simulink model "Scenario_Analysis_Simu"  (R2023b)
settings: Solver=VariableStepAuto  StartTime=0.0  StopTime=1  RelTol=1e-3
values from neighbouring files (symbols this model uses):
  X_init = P.X(1)    [Scenario_Analysis_Main.m]
  X_pos = P.X(i)    [Scenario_Analysis_Main.m]
  Y_init = P.Y(1)    [Scenario_Analysis_Main.m]
  Y_pos = P.Y(i)    [Scenario_Analysis_Main.m]
  Z_init = P.Z(1)    [Scenario_Analysis_Main.m]
  Z_pos = P.Z(i)    [Scenario_Analysis_Main.m]
settings Model: Creator=Dell  LastModifiedBy=Dell

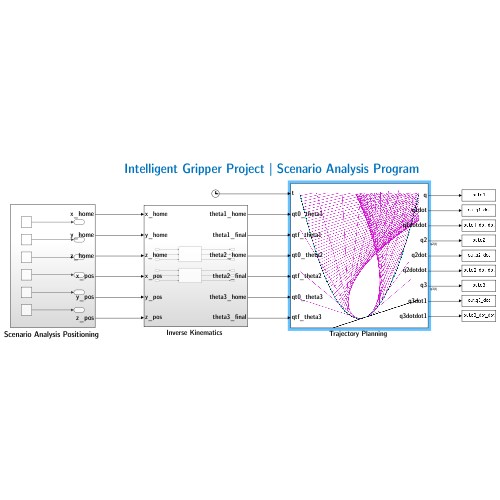
[thumbnail: Simulink's stored preview of the top-level diagram]
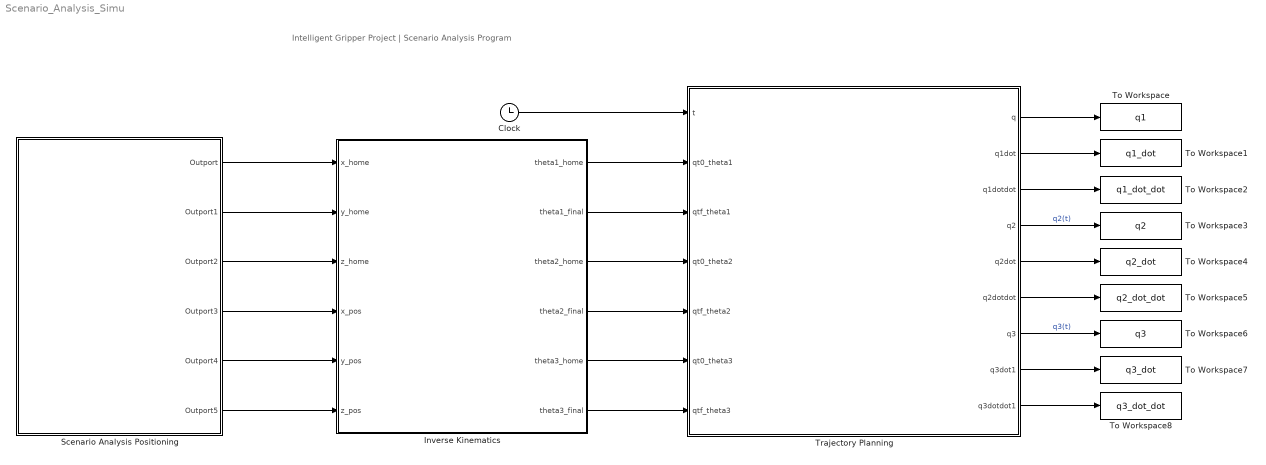
== system Scenario_Analysis_Simu ==
  note: Intelligent Gripper Project | Scenario Analysis Program
  Clock : Clock
      settings: Decimation=5
  "Inverse Kinematics " : Subsystem
  "Scenario Analysis Positioning " : Subsystem
  To Workspace : ToWorkspace  VariableName=q1  SampleTime=-1
  To Workspace1 : ToWorkspace  VariableName=q1_dot  SampleTime=-1
  To Workspace2 : ToWorkspace  VariableName=q1_dot_dot  SampleTime=-1
  To Workspace3 : ToWorkspace  VariableName=q2  SampleTime=-1
  To Workspace4 : ToWorkspace  VariableName=q2_dot  SampleTime=-1
  To Workspace5 : ToWorkspace  VariableName=q2_dot_dot  SampleTime=-1
  To Workspace6 : ToWorkspace  VariableName=q3  SampleTime=-1
  To Workspace7 : ToWorkspace  VariableName=q3_dot  SampleTime=-1
  To Workspace8 : ToWorkspace  VariableName=q3_dot_dot  SampleTime=-1
  "Trajectory Planning " : Subsystem
      mask Display: image('kisspng-caustic-tschirnhausen-cubic-curve-nephroid-parabol-caustique-wikipdia-5c6cdcbe1d93b4.9550090715506382701212.png');
  wires:
  "Inverse Kinematics "/5(theta3_home) -> "Trajectory Planning "/6(qt0_theta3)
  "Scenario Analysis Positioning "/2(Outport1) -> "Inverse Kinematics "/2(y_home)
  "Scenario Analysis Positioning "/3(Outport2) -> "Inverse Kinematics "/3(z_home)
  "Inverse Kinematics "/1(theta1_home) -> "Trajectory Planning "/2(qt0_theta1)
  "Inverse Kinematics "/2(theta1_final) -> "Trajectory Planning "/3(qtf_theta1)
  "Scenario Analysis Positioning "/1(Outport) -> "Inverse Kinematics "/1(x_home)
  "Inverse Kinematics "/6(theta3_final) -> "Trajectory Planning "/7(qtf_theta3)
  "Inverse Kinematics "/4(theta2_final) -> "Trajectory Planning "/5(qtf_theta2)
  "Scenario Analysis Positioning "/6(Outport5) -> "Inverse Kinematics "/6(z_pos)
  "Inverse Kinematics "/3(theta2_home) -> "Trajectory Planning "/4(qt0_theta2)
  "Scenario Analysis Positioning "/5(Outport4) -> "Inverse Kinematics "/5(y_pos)
  "Scenario Analysis Positioning "/4(Outport3) -> "Inverse Kinematics "/4(x_pos)
  Clock/1 -> "Trajectory Planning "/1(t)
  "Trajectory Planning "/1(q) -> To Workspace/1
  "Trajectory Planning "/2(q1dot) -> To Workspace1/1
  "Trajectory Planning "/3(q1dotdot) -> To Workspace2/1
  "Trajectory Planning "/4(q2) -> To Workspace3/1  "q2(t)"
  "Trajectory Planning "/5(q2dot) -> To Workspace4/1
  "Trajectory Planning "/6(q2dotdot) -> To Workspace5/1
  "Trajectory Planning "/7(q3) -> To Workspace6/1  "q3(t)"
  "Trajectory Planning "/8(q3dot1) -> To Workspace7/1
  "Trajectory Planning "/9(q3dotdot1) -> To Workspace8/1

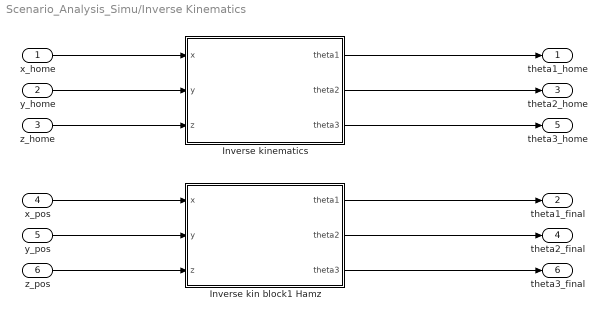
== system Scenario_Analysis_Simu/Inverse Kinematics  ==
  x_home : Inport
  y_home : Inport  Port=2
  z_home : Inport  Port=3
  x_pos : Inport  Port=4
  y_pos : Inport  Port=5
  z_pos : Inport  Port=6
  "Inverse kin block1 Hamz " : MATLAB Function  TreatAsAtomicUnit=on
  Inverse kinematics : MATLAB Function  TreatAsAtomicUnit=on
  theta1_home : Outport
  theta1_final : Outport  Port=2
  theta2_home : Outport  Port=3
  theta2_final : Outport  Port=4
  theta3_home : Outport  Port=5
  theta3_final : Outport  Port=6
  wires:
  z_home/1 -> Inverse kinematics/3(z)
  "Inverse kin block1 Hamz "/3(theta3) -> theta3_final/1
  y_home/1 -> Inverse kinematics/2(y)
  Inverse kinematics/1(theta1) -> theta1_home/1
  Inverse kinematics/3(theta3) -> theta3_home/1
  "Inverse kin block1 Hamz "/2(theta2) -> theta2_final/1
  x_home/1 -> Inverse kinematics/1(x)
  x_pos/1 -> "Inverse kin block1 Hamz "/1(x)
  Inverse kinematics/2(theta2) -> theta2_home/1
  y_pos/1 -> "Inverse kin block1 Hamz "/2(y)
  z_pos/1 -> "Inverse kin block1 Hamz "/3(z)
  "Inverse kin block1 Hamz "/1(theta1) -> theta1_final/1

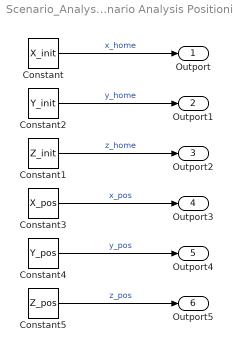
== system Scenario_Analysis_Simu/Scenario Analysis Positioning  ==
  Constant : Constant  Value=X_init
  Constant1 : Constant  Value=Z_init
  Constant2 : Constant  Value=Y_init
  Constant3 : Constant  Value=X_pos
  Constant4 : Constant  Value=Y_pos
  Constant5 : Constant  Value=Z_pos
  Outport : Outport
  Outport1 : Outport  Port=2
  Outport2 : Outport  Port=3
  Outport3 : Outport  Port=4
  Outport4 : Outport  Port=5
  Outport5 : Outport  Port=6
  wires:
  Constant/1 -> Outport/1  "x_home"
  Constant2/1 -> Outport1/1  "y_home"
  Constant3/1 -> Outport3/1  "x_pos"
  Constant4/1 -> Outport4/1  "y_pos"
  Constant5/1 -> Outport5/1  "z_pos"
  Constant1/1 -> Outport2/1  "z_home"

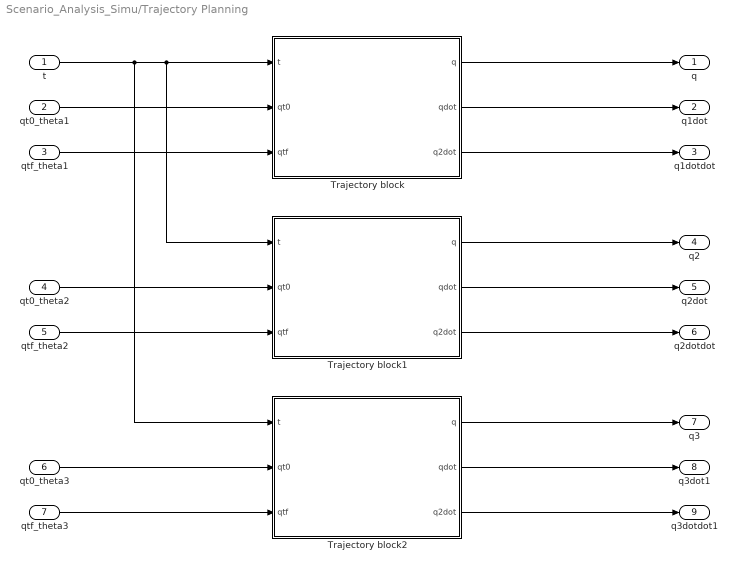
== system Scenario_Analysis_Simu/Trajectory Planning  ==
  t : Inport
  qt0_theta1 : Inport  Port=2
  qtf_theta1 : Inport  Port=3
  qt0_theta2 : Inport  Port=4
  qtf_theta2 : Inport  Port=5
  qt0_theta3 : Inport  Port=6
  qtf_theta3 : Inport  Port=7
  Trajectory block : MATLAB Function  TreatAsAtomicUnit=on
  Trajectory block1 : MATLAB Function  TreatAsAtomicUnit=on
  Trajectory block2 : MATLAB Function  TreatAsAtomicUnit=on
  q : Outport
  q1dot : Outport  Port=2
  q1dotdot : Outport  Port=3
  q2 : Outport  Port=4
  q2dot : Outport  Port=5
  q2dotdot : Outport  Port=6
  q3 : Outport  Port=7
  q3dot1 : Outport  Port=8
  q3dotdot1 : Outport  Port=9
  wires:
  qt0_theta1/1 -> Trajectory block/2(qt0)
  qtf_theta1/1 -> Trajectory block/3(qtf)
  qt0_theta2/1 -> Trajectory block1/2(qt0)
  qtf_theta2/1 -> Trajectory block1/3(qtf)
  t/1 -> Trajectory block2/1(t), Trajectory block1/1(t), Trajectory block/1(t)
  qt0_theta3/1 -> Trajectory block2/2(qt0)
  qtf_theta3/1 -> Trajectory block2/3(qtf)
  Trajectory block/1(q) -> q/1
  Trajectory block/2(qdot) -> q1dot/1
  Trajectory block/3(q2dot) -> q1dotdot/1
  Trajectory block1/1(q) -> q2/1
  Trajectory block1/2(qdot) -> q2dot/1
  Trajectory block1/3(q2dot) -> q2dotdot/1
  Trajectory block2/1(q) -> q3/1
  Trajectory block2/2(qdot) -> q3dot1/1
  Trajectory block2/3(q2dot) -> q3dotdot1/1

== matlab function Scenario_Analysis_Simu/Inverse Kinematics /Inverse kinematics ==
  data: x input; theta1 output; y input; z input; theta2 output; theta3 output
function [theta1,theta2,theta3] = inverse_kin(x,y,z)
%% calling get-thetas function
%Some delta robot dimensions & constants
SB = 280;    % base side length
SP = 90;    % platform side length
L  = 250;    % driver link length
l  = 500;    % driven link length
delta = 69;  % distance between the each pair of driven links
tau = 100;   % distance between the bearing of the driver link's revolute joint

max_beta = pi/6;   % max angle for the spherical joints
min_angle = -pi/6;  % the minimum angle allowed for the motors
max_angle = pi/3;  % the maximum angle allowed for the motors

wB = (SB*sqrt(3))/(6);
uB = (SB*sqrt(3))/(3);
wP = (SP*sqrt(3))/(6);
uP = (SP*sqrt(3))/(3);

delta_2 = delta/2;
tau_2 = tau/2;

a = wB-uP;
b = (SP-sqrt(3)*wB)/2;
c = wP-0.5*wB;
%constants;
F  = 2*z*L;
% Getting theta 1:
    E_1 = 2*L*(y+a);
    G_1 = x*x + y*y + z*z + a*a + L*L + 2*y*a - l*l;
t_plus1 = (-F + sqrt(((E_1)^2)+((F)^2)-((G_1)^2)))/(G_1-E_1);
t_minus1 = (-F - sqrt(((E_1)^2)+((F)^2)-((G_1)^2)))/(G_1-E_1);
if (abs(t_plus1)>abs(t_minus1))
  t1=t_minus1;
else
  t1=t_plus1;
end
theta1 = 2*atan(t1);
% Getting theta 2:
    E_2 = -L*(sqrt(3)*(x+b)+y+c);
    G_2 = x*x + y*y + z*z + b*b + c*c + L*L + 2*(x*b + y*c) - l*l;
t_plus2 = (-F + sqrt(((E_2)^2)+((F)^2)-((G_2)^2)))/(G_2-E_2);
t_minus2 = (-F - sqrt(((E_2)^2)+((F)^2)-((G_2)^2)))/(G_2-E_2);
if (abs(t_plus2)>abs(t_minus2))
  t2=t_minus2;
else
  t2=t_plus2;
end
theta2 = 2*atan(t2);
% Getting theta 3:
    E_3 = L*(sqrt(3)*(x-b)-y-c);
    G_3 = x*x + y*y + z*z + b*b + c*c + L*L + 2*(-x*b + y*c) - l*l;
t_plus3 = (-F + sqrt(((E_3)^2)+((F)^2)-((G_3)^2)))/(G_3-E_3);
t_minus3 = (-F - sqrt(((E_3)^2)+((F)^2)-((G_3)^2)))/(G_3-E_3);
if (abs(t_plus3)>abs(t_minus3))
  t3=t_minus3;
else
  t3=t_plus3;
end
theta3 = 2*atan(t3);
% saving the three thetas in thetas array

end
%%

== matlab function Scenario_Analysis_Simu/Trajectory Planning /Trajectory block ==
  data: q output; qdot output; q2dot output; t input; qt0 input; qtf input
function [q,qdot,q2dot] = trajectory_planning(t,qt0,qtf)
t0=0;
tf=1;
%qt0=-2*pi/6;
%qtf=pi/6;
qdott0=0;
qdottf=0;

A=[1 t0  t0^2 t0^3;0 1 2*t0 3*t0^2;1 tf tf^2 tf^3;0 1 2*tf 3*tf^2];
RHS=[qt0;qdott0;qtf;qdottf];

coeffs=inv(A)*RHS;

%t=linspace(t0,tf,100);
q=coeffs(4)*t.^3+coeffs(3)*t.^2+coeffs(2)*t+coeffs(1);
qdot=3*coeffs(4)*t.^2+2*coeffs(3)*t+coeffs(2);
q2dot=6*coeffs(4)*t+2*coeffs(3);

== matlab function Scenario_Analysis_Simu/Inverse Kinematics /Inverse kin block1 Hamz  ==
  data: x input; theta1 output; y input; z input; theta2 output; theta3 output
function [theta1,theta2,theta3] = inverse_kin(x,y,z)
%% Entering coords of end-effector 
%x = input("Enter X position of end effector :");
%y = input("Enter Y position of end effector :");
%z = input("Enter Z position of end effector :");
%% calling get-thetas function
%Some delta robot dimensions & constants
SB = 280;    % base side length
SP = 90;    % platform side length
L  = 250;    % driver link length
l  = 500;    % driven link length
delta = 69;  % distance between the each pair of driven links
tau = 100;   % distance between the bearing of the driver link's revolute joint

max_beta = pi/6;   % max angle for the spherical joints
min_angle = -pi/6;  % the minimum angle allowed for the motors
max_angle = pi/3;  % the maximum angle allowed for the motors

wB = (SB*sqrt(3))/(6);
uB = (SB*sqrt(3))/(3);
wP = (SP*sqrt(3))/(6);
uP = (SP*sqrt(3))/(3);

delta_2 = delta/2;
tau_2 = tau/2;

a = wB-uP;
b = (SP-sqrt(3)*wB)/2;
c = wP-0.5*wB;
%constants;
F  = 2*z*L;
% Getting theta 1:
    E_1 = 2*L*(y+a);
    G_1 = x*x + y*y + z*z + a*a + L*L + 2*y*a - l*l;
t_plus1 = (-F + sqrt(((E_1)^2)+((F)^2)-((G_1)^2)))/(G_1-E_1);
t_minus1 = (-F - sqrt(((E_1)^2)+((F)^2)-((G_1)^2)))/(G_1-E_1);
if (abs(t_plus1)>abs(t_minus1))
  t1=t_minus1;
else
  t1=t_plus1;
end
theta1 = 2*atan(t1);
% Getting theta 2:
    E_2 = -L*(sqrt(3)*(x+b)+y+c);
    G_2 = x*x + y*y + z*z + b*b + c*c + L*L + 2*(x*b + y*c) - l*l;
t_plus2 = (-F + sqrt(((E_2)^2)+((F)^2)-((G_2)^2)))/(G_2-E_2);
t_minus2 = (-F - sqrt(((E_2)^2)+((F)^2)-((G_2)^2)))/(G_2-E_2);
if (abs(t_plus2)>abs(t_minus2))
  t2=t_minus2;
else
  t2=t_plus2;
end
theta2 = 2*atan(t2);
% Getting theta 3:
    E_3 = L*(sqrt(3)*(x-b)-y-c);
    G_3 = x*x + y*y + z*z + b*b + c*c + L*L + 2*(-x*b + y*c) - l*l;
t_plus3 = (-F + sqrt(((E_3)^2)+((F)^2)-((G_3)^2)))/(G_3-E_3);
t_minus3 = (-F - sqrt(((E_3)^2)+((F)^2)-((G_3)^2)))/(G_3-E_3);
if (abs(t_plus3)>abs(t_minus3))
  t3=t_minus3;
else
  t3=t_plus3;
end
theta3 = 2*atan(t3);
% saving the three thetas in thetas array

end
%%

== matlab function Scenario_Analysis_Simu/Trajectory Planning /Trajectory block1 ==
  data: q output; qdot output; q2dot output; t input; qt0 input; qtf input
function [q,qdot,q2dot] = trajectory_planning(t,qt0,qtf)
t0=0;
tf=1;
%qt0=-2*pi/6;
%qtf=pi/6;
qdott0=0;
qdottf=0;

A=[1 t0  t0^2 t0^3;0 1 2*t0 3*t0^2;1 tf tf^2 tf^3;0 1 2*tf 3*tf^2];
RHS=[qt0;qdott0;qtf;qdottf];

coeffs=inv(A)*RHS;

%t=linspace(t0,tf,100);
q=coeffs(4)*t.^3+coeffs(3)*t.^2+coeffs(2)*t+coeffs(1);
qdot=3*coeffs(4)*t.^2+2*coeffs(3)*t+coeffs(2);
q2dot=6*coeffs(4)*t+2*coeffs(3);

== matlab function Scenario_Analysis_Simu/Trajectory Planning /Trajectory block2 ==
  data: q output; qdot output; q2dot output; t input; qt0 input; qtf input
function [q,qdot,q2dot] = trajectory_planning(t,qt0,qtf)
t0=0;
tf=1;
%qt0=-2*pi/6;
%qtf=pi/6;
qdott0=0;
qdottf=0;

A=[1 t0  t0^2 t0^3;0 1 2*t0 3*t0^2;1 tf tf^2 tf^3;0 1 2*tf 3*tf^2];
RHS=[qt0;qdott0;qtf;qdottf];

coeffs=inv(A)*RHS;

%t=linspace(t0,tf,100);
q=coeffs(4)*t.^3+coeffs(3)*t.^2+coeffs(2)*t+coeffs(1);
qdot=3*coeffs(4)*t.^2+2*coeffs(3)*t+coeffs(2);
q2dot=6*coeffs(4)*t+2*coeffs(3);
